simulink model "linear_ss_control"  (R2019b)
settings: Solver=ode45  StartTime=0.0  StopTime=700.0  MaxStep=0.01  RelTol=1e-8
settings Model: Creator=Hector  LastModifiedBy=Hector

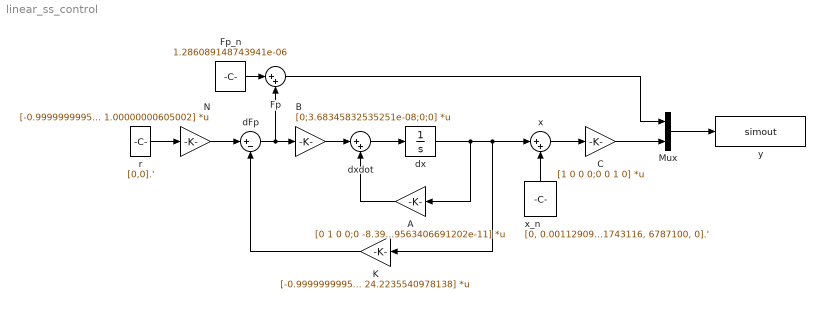
== system linear_ss_control ==
  A : Gain  Gain=[0 1 0 0;0 -8.39126813382404e-11 -1.39595873998803e-20 -3.3271699050138e-10;0 0 0 1;0 15326.5171394046 3.8245444931179e-06 -4.19563406691202e-11]  Multiplication=Matrix(K*u)
  B : Gain  Gain=[0;3.68345832535251e-08;0;0]  Multiplication=Matrix(K*u)
  C : Gain  Gain=[1 0 0 0;0 0 1 0]  Multiplication=Matrix(K*u)
  Fp : Sum  Inputs=|++
  Fp_n : Constant  Value=1.286089148743941e-06
  K : Gain  Gain=[-0.999999999517925 4489802.13130477 1.00112038113525 24.2235540978138]  Multiplication=Matrix(K*u)
  Mux : Mux  Inputs=2
  N : Gain  Gain=[-0.999999999517925 1.00000000605002]  Multiplication=Matrix(K*u)
  dFp : Sum  Inputs=|+-
  dx : Integrator  InitialCondition=[0, 0, -1*10^-6, 0].'
  dxdot : Sum  Inputs=|++
  r : Constant  Value=[0,0].'
  x : Sum  Inputs=|++
  x_n : Constant  Value=[0, 0.001129091743116, 6787100, 0].'
  y : ToWorkspace  VariableName=simout  SaveFormat=Timeseries  SampleTime=-1
  wires:
  dx/1 -> x/1, K/1, A/1
  dxdot/1 -> dx/1
  A/1 -> dxdot/2
  x/1 -> C/1
  x_n/1 -> x/2
  B/1 -> dxdot/1
  K/1 -> dFp/2
  Fp_n/1 -> Fp/1
  dFp/1 -> B/1, Fp/2
  N/1 -> dFp/1
  Mux/1 -> y/1
  C/1 -> Mux/2
  Fp/1 -> Mux/1
  r/1 -> N/1
